simulink model "chap5_6sim"  (Simulink 3.00)
settings: Solver=ode45  StartTime=0.0  StopTime=10  RelTol=1e-3
settings Model: LastModifiedBy=liu

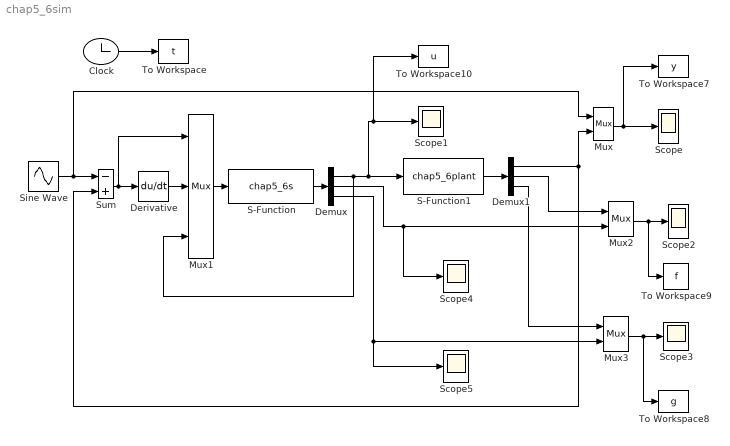
== system chap5_6sim ==
  Clock : Clock
  Demux : Demux  Outputs=3
  Demux1 : Demux  Outputs=3
  Derivative : Derivative
  Mux : Mux  Inputs=2
      settings: DisplayOption=none
  Mux1 : Mux  Inputs=3
      settings: DisplayOption=none
  Mux2 : Mux  Inputs=2
      settings: DisplayOption=none
  Mux3 : Mux  Inputs=2
      settings: DisplayOption=none
  S-Function : S-Function  FunctionName=chap5_6s  PortCounts=[]  SFunctionModules=''
  S-Function1 : S-Function  FunctionName=chap5_6plant  PortCounts=[]  SFunctionModules=''
  Scope{,1..5} (6 alike) : Scope
      Scope settings: TimeRange=3  YMin=-0.1  YMax=0.09  SaveToWorkspace=off  SaveName=ScopeData  MaxRows=500000
      Scope1 settings: TimeRange=3  YMin=-5.5  YMax=3  SaveToWorkspace=off  SaveName=ScopeData  MaxRows=500000
      Scope2 settings: TimeRange=3  YMin=-0.1  YMax=1  SaveToWorkspace=off  SaveName=ScopeData  MaxRows=500000
      Scope3 settings: TimeRange=3  YMin=-0.1  YMax=0.1  SaveToWorkspace=off  SaveName=ScopeData  MaxRows=500000
      Scope4 settings: TimeRange=3  YMin=-0.1  YMax=0.1  SaveToWorkspace=off  SaveName=ScopeData  MaxRows=500000
      Scope5 settings: TimeRange=3  YMin=-0.1  YMax=0.1  SaveToWorkspace=off  SaveName=ScopeData  MaxRows=500000
  Sine Wave : Sin  Amplitude=0.10  Frequency=pi  Phase=0  SampleTime=0
  Sum : Sum  Inputs=-+  SaturateOnIntegerOverflow=on
  To Workspace : ToWorkspace  VariableName=t  SampleTime=-1  SaveFormat=Matrix
  To Workspace10 : ToWorkspace  VariableName=u  SampleTime=-1  SaveFormat=Matrix
  To Workspace7 : ToWorkspace  VariableName=y  SampleTime=-1  SaveFormat=Matrix
  To Workspace8 : ToWorkspace  VariableName=g  SampleTime=-1  SaveFormat=Matrix
  To Workspace9 : ToWorkspace  VariableName=f  SampleTime=-1  SaveFormat=Matrix
  wires:
  Mux1/1 -> S-Function/1
  S-Function/1 -> Demux/1
  S-Function1/1 -> Demux1/1
  Demux1/1 -> Sum/2, Mux/2
  Sum/1 -> Mux1/1, Derivative/1
  Derivative/1 -> Mux1/2
  Demux1/3 -> Mux3/1
  Demux/3 -> Mux3/2, Scope5/1
  Demux/2 -> Mux2/2, Scope4/1
  Demux/1 -> S-Function1/1, Scope1/1, To Workspace10/1, Mux1/3
  Mux/1 -> Scope/1, To Workspace7/1
  Demux1/2 -> Mux2/1
  Mux3/1 -> Scope3/1, To Workspace8/1
  Mux2/1 -> Scope2/1, To Workspace9/1
  Sine Wave/1 -> Sum/1, Mux/1
  Clock/1 -> To Workspace/1
